simulink model "modelcompare"  (R2025b)
settings: Solver=VariableStepAuto  StartTime=0.0  StopTime=1296  RelTol=1e-3
(part 2 of 2)

== system modelcompare/Cooling Jacket Model4/Water to out ==
  Th : Inport
  mdot : Inport  Port=2
  Cpw : Inport  Port=3
  Mw : Inport  Port=4
  T_in : Inport  Port=5
  A : Inport  Port=6
  hw : Inport  Port=7
  Integrator2 : Integrator  InitialCondition=35
  MATLAB Function2 : MATLAB Function  TreatAsAtomicUnit=on
  Tout : Outport
  wires:
  Integrator2/1 -> Tout/1, MATLAB Function2/2(Tout)
  MATLAB Function2/1(dTout) -> Integrator2/1
  Th/1 -> MATLAB Function2/1(Th)
  T_in/1 -> MATLAB Function2/6(T_in)
  Mw/1 -> MATLAB Function2/3(Mw)
  mdot/1 -> MATLAB Function2/5(mdot)
  Cpw/1 -> MATLAB Function2/4(Cpw)
  A/1 -> MATLAB Function2/7(A)
  hw/1 -> MATLAB Function2/8(hw)

== system modelcompare/Cooling Jacket Model4/housing to water ==
  Ts : Inport
  k : Inport  Port=2
  d : Inport  Port=3
  Mh : Inport  Port=4
  Cph : Inport  Port=5
  A_sh : Inport  Port=6
  h : Inport  Port=7
  Tout : Inport  Port=8
  A_hw : Inport  Port=9
  Integrator1 : Integrator  InitialCondition=35
  MATLAB Function1 : MATLAB Function  TreatAsAtomicUnit=on
  Surface Temperature : Outport
  wires:
  MATLAB Function1/1(dTh) -> Integrator1/1
  k/1 -> MATLAB Function1/4(k)
  Ts/1 -> MATLAB Function1/1(Ts)
  Tout/1 -> MATLAB Function1/3(Tin)
  Integrator1/1 -> MATLAB Function1/2(Th), Surface Temperature/1
  d/1 -> MATLAB Function1/10(d_sh)
  Cph/1 -> MATLAB Function1/9(C_ph)
  Mh/1 -> MATLAB Function1/8(M_h)
  A_hw/1 -> MATLAB Function1/6(A_hw)
  A_sh/1 -> MATLAB Function1/5(A_sh)
  h/1 -> MATLAB Function1/7(h)

== matlab function modelcompare/Cooling Jacket Model2/MATLAB Function ==
  data: mdot input; h output; D input; CSA input; k input; f input; Pr input; Nu output; Re output; V output
function [h, Nu, Re, V]= fcn(mdot, D, CSA, k, f, Pr)
V = mdot/(1000*CSA);
Re = (V*1000*D)/0.00089;
Nu = ((f/8)*(Re-1000)*Pr)/(1+(12.7*(f/8)^0.5 * (Pr^(2/3) - 1)));
h = (Nu*k)/D;
end

== matlab function modelcompare/Battery Capacity/MATLAB Function ==
  data: Capacity output; energy input
function Capacity = fcn(energy)
    Capacity = energy/(12*3600);
end

== matlab function modelcompare/Battery Capacity1/MATLAB Function ==
  data: Capacity output; energy input
function Capacity = fcn(energy)
    Capacity = energy/(12*3600);
end

== matlab function modelcompare/Cooling Jacket Model1/MATLAB Function ==
  data: mdot input; h output; D input; CSA input; k input; f input; Pr input; Nu output; Re output; V output
function [h, Nu, Re, V]= fcn(mdot, D, CSA, k, f, Pr)
V = mdot/(1000*CSA);
Re = (V*1000*D)/0.00089;
Nu = ((f/8)*(Re-1000)*Pr)/(1+(12.7*(f/8)^0.5 * (Pr^(2/3) - 1)));
h = (Nu*k)/D;
end

== matlab function modelcompare/Cooling Jacket Model2/Stator to Housing/MATLAB Function ==
  data: Q_gen input; Ts input; dTs output; Th input; Ms input; Cps input; k input; A input; d input
function dTs = f1(Q_gen, Ts, Th, Ms, Cps, k, A, d)
    dTs = (Q_gen - (Ts - Th) * k * A / d) / (Ms * Cps);
end

== matlab function modelcompare/Cooling Jacket Model2/Water to out/MATLAB Function2 ==
  data: Th input; Tout input; Mw input; Cpw input; mdot input; T_in input; dTout output; A input; hw input
function dTout = f3(Th, Tout, Mw, Cpw, mdot, T_in, A, hw)
    q_from_housing = (Th - Tout) * hw * A;
    q_out = (Tout - T_in) * mdot * Cpw;
    dTout = ((q_from_housing - q_out)) / (Mw * Cpw);
end

== matlab function modelcompare/Cooling Jacket Model2/housing to water/MATLAB Function1 ==
  data: Ts input; Th input; Tin input; k input; A_sh input; A_hw input; dTh output; h input; M_h input; C_ph input; d_sh input
function dTh = f2(Ts, Th, Tin, k, A_sh, A_hw, h, M_h, C_ph, d_sh)
    dTh = ((k*A_sh*(Ts - Th)/d_sh) - h*A_hw*(Th - Tin)) / (M_h * C_ph);
end

== matlab function modelcompare/Cooling Jacket Model1/Stator to Housing/MATLAB Function ==
  data: Q_gen input; Ts input; dTs output; Th input; Ms input; Cps input; k input; A input; d input
function dTs = f1(Q_gen, Ts, Th, Ms, Cps, k, A, d)
    dTs = (Q_gen - (Ts - Th) * k * A / d) / (Ms * Cps);
end

== matlab function modelcompare/Cooling Jacket Model1/Water to out/MATLAB Function2 ==
  data: Th input; Tout input; Mw input; Cpw input; mdot input; T_in input; dTout output; A input; hw input
function dTout = f3(Th, Tout, Mw, Cpw, mdot, T_in, A, hw)
    q_from_housing = (Th - Tout) * hw * A;
    q_out = (Tout - T_in) * mdot * Cpw;
    dTout = ((q_from_housing - q_out)) / (Mw * Cpw);
end

== matlab function modelcompare/Cooling Jacket Model1/housing to water/MATLAB Function1 ==
  data: Ts input; Th input; Tin input; k input; A_sh input; A_hw input; dTh output; h input; M_h input; C_ph input; d_sh input
function dTh = f2(Ts, Th, Tin, k, A_sh, A_hw, h, M_h, C_ph, d_sh)
    dTh = ((k*A_sh*(Ts - Th)/d_sh) - h*A_hw*(Th - Tin)) / (M_h * C_ph);
end

== matlab function modelcompare/Pump Controller1/MATLAB Function ==
  data: StatorTemp input; mdot output; maximumFlowRate input; TempThreshold input
function mdot = fcn(StatorTemp, maximumFlowRate, TempThreshold)
if StatorTemp < 80 && StatorTemp > TempThreshold
    mdot = ((StatorTemp-TempThreshold)/(80 - TempThreshold))*maximumFlowRate;
elseif StatorTemp < TempThreshold
    mdot = 0;
else
    mdot = maximumFlowRate;
end
end

== matlab function modelcompare/Pump Controller1/MATLAB Function1 ==
  data: mdot input; power output; maxMdot input; maxcurrent input
function power = fcn(mdot, maxMdot, maxcurrent)
    power = (((4-maxcurrent)/(0-maxMdot))*(mdot - maxMdot) + maxcurrent)*12;
end

== matlab function modelcompare/Radiator1/MATLAB Function ==
  data: K input; h_wr output; D input; mdot input; A input
function h_wr = fcn(K, D, mdot, A)
Vm = mdot/(A * 24 * 1000);
Nu = 0.023 * (((1000*D*Vm)/0.001002)^0.8) * (6.9^0.4);
h_wr = (Nu * K)/D;
end

== matlab function modelcompare/Radiator1/MATLAB Function1 ==
  data: K input; h_ar output; D input; Va input
function h_ar = fcn(K, D, Va)
Nu = 0.664*((Va*D)/0.0000148)^0.5*(0.71)^0.33;
h_ar = (Nu * K)/D;
end

== matlab function modelcompare/Radiator1/Radiator to Air ==
  data: Trad input; Tair input; dTair output; A input; h input; v_air input; c_air input; m_air input; T_amb input; rho_air input
function dTair = f2(Trad, Tair, A, h, v_air, c_air, m_air, T_amb, rho_air)
    dTair = ((Trad - Tair) * h * A - (Tair - T_amb) * v_air * rho_air * A * c_air) / (m_air * c_air);
end

== matlab function modelcompare/Pump Controller/MATLAB Function1 ==
  data: mdot input; power output; maxMdot input; maxcurrent input
function power = fcn(mdot, maxMdot, maxcurrent)
    power = (((4-maxcurrent)/(0-maxMdot))*(mdot - maxMdot) + maxcurrent)*12;
end

== matlab function modelcompare/Radiator1/Water ==
  data: Tout_water input; T_in_water input; Trad input; dTout_water output; mdot_w input; c_w input; h_wr input; A_wr input; m_w_rad input
function dTout_water = f3(Tout_water, T_in_water, Trad, mdot_w, c_w, h_wr, A_wr, m_w_rad)
    dTout_water = ((T_in_water - Tout_water) * mdot_w * c_w - (Tout_water - Trad) * h_wr * A_wr) / (m_w_rad * c_w);
end

== matlab function modelcompare/Radiator1/Water to Radiator ==
  data: Trad input; Tair input; dTrad output; Tout_water input; h_wr input; A_wr input; h input; A input; m_rad input; c_rad input
function dTrad = f1(Trad, Tair, Tout_water, h_wr, A_wr, h, A, m_rad, c_rad)
    dTrad = ((Tout_water - Trad) * h_wr * A_wr - (Trad - Tair) * h * A) / (m_rad * c_rad);
end

== matlab function modelcompare/Battery Capacity3/MATLAB Function ==
  data: Capacity output; energy input
function Capacity = fcn(energy)
    Capacity = energy/(12*3600);
end

== matlab function modelcompare/Cooling Jacket Model4/MATLAB Function ==
  data: mdot input; h output; D input; CSA input; k input; f input; Pr input; Nu output; Re output; V output
function [h, Nu, Re, V]= fcn(mdot, D, CSA, k, f, Pr)
V = mdot/(1000*CSA);
Re = (V*1000*D)/0.00089;
Nu = ((f/8)*(Re-1000)*Pr)/(1+(12.7*(f/8)^0.5 * (Pr^(2/3) - 1)));
h = (Nu*k)/D;
end

== matlab function modelcompare/Cooling Jacket Model4/Stator to Housing/MATLAB Function ==
  data: Q_gen input; Ts input; dTs output; Th input; Ms input; Cps input; k input; A input; d input
function dTs = f1(Q_gen, Ts, Th, Ms, Cps, k, A, d)
    dTs = (Q_gen - (Ts - Th) * k * A / d) / (Ms * Cps);
end

== matlab function modelcompare/Cooling Jacket Model4/Water to out/MATLAB Function2 ==
  data: Th input; Tout input; Mw input; Cpw input; mdot input; T_in input; dTout output; A input; hw input
function dTout = f3(Th, Tout, Mw, Cpw, mdot, T_in, A, hw)
    q_from_housing = (Th - Tout) * hw * A;
    q_out = (Tout - T_in) * mdot * Cpw;
    dTout = ((q_from_housing - q_out)) / (Mw * Cpw);
end

== matlab function modelcompare/Cooling Jacket Model4/housing to water/MATLAB Function1 ==
  data: Ts input; Th input; Tin input; k input; A_sh input; A_hw input; dTh output; h input; M_h input; C_ph input; d_sh input
function dTh = f2(Ts, Th, Tin, k, A_sh, A_hw, h, M_h, C_ph, d_sh)
    dTh = ((k*A_sh*(Ts - Th)/d_sh) - h*A_hw*(Th - Tin)) / (M_h * C_ph);
end

== matlab function modelcompare/Pump Controller/MATLAB Function ==
  data: mdot output
function mdot = fcn()

    mdot = 0.15;

end

== matlab function modelcompare/Pump Controller3/MATLAB Function1 ==
  data: mdot input; power output; maxMdot input; maxcurrent input
function power = fcn(mdot, maxMdot, maxcurrent)
    power = (((4-maxcurrent)/(0-maxMdot))*(mdot - maxMdot) + maxcurrent)*12;
end

== matlab function modelcompare/Radiator3/MATLAB Function ==
  data: K input; h_wr output; D input; mdot input; A input
function h_wr = fcn(K, D, mdot, A)
Vm = mdot/(A * 24 * 1000);
Nu = 0.023 * (((1000*D*Vm)/0.001002)^0.8) * (6.9^0.4);
h_wr = (Nu * K)/D;
end

== matlab function modelcompare/Radiator3/MATLAB Function1 ==
  data: K input; h_ar output; D input; Va input
function h_ar = fcn(K, D, Va)
Nu = 0.664*((Va*D)/0.0000148)^0.5*(0.71)^0.33;
h_ar = (Nu * K)/D;
end

== matlab function modelcompare/Radiator3/Radiator to Air ==
  data: Trad input; Tair input; dTair output; A input; h input; v_air input; c_air input; m_air input; T_amb input; rho_air input
function dTair = f2(Trad, Tair, A, h, v_air, c_air, m_air, T_amb, rho_air)
    dTair = ((Trad - Tair) * h * A - (Tair - T_amb) * v_air * rho_air * A * c_air) / (m_air * c_air);
end

== matlab function modelcompare/Radiator3/Water ==
  data: Tout_water input; T_in_water input; Trad input; dTout_water output; mdot_w input; c_w input; h_wr input; A_wr input; m_w_rad input
function dTout_water = f3(Tout_water, T_in_water, Trad, mdot_w, c_w, h_wr, A_wr, m_w_rad)
    dTout_water = ((T_in_water - Tout_water) * mdot_w * c_w - (Tout_water - Trad) * h_wr * A_wr) / (m_w_rad * c_w);
end

== matlab function modelcompare/Radiator/MATLAB Function ==
  data: K input; h_wr output; D input; mdot input; A input
function h_wr = fcn(K, D, mdot, A)
Vm = mdot/(A * 24 * 1000);
Nu = 0.023 * (((1000*D*Vm)/0.001002)^0.8) * (6.9^0.4);
h_wr = (Nu * K)/D;
end

== matlab function modelcompare/Radiator3/Water to Radiator ==
  data: Trad input; Tair input; dTrad output; Tout_water input; h_wr input; A_wr input; h input; A input; m_rad input; c_rad input
function dTrad = f1(Trad, Tair, Tout_water, h_wr, A_wr, h, A, m_rad, c_rad)
    dTrad = ((Tout_water - Trad) * h_wr * A_wr - (Trad - Tair) * h * A) / (m_rad * c_rad);
end

== matlab function modelcompare/Radiator/Water to Radiator ==
  data: Trad input; Tair input; dTrad output; Tout_water input; h_wr input; A_wr input; h input; A input; m_rad input; c_rad input
function dTrad = f1(Trad, Tair, Tout_water, h_wr, A_wr, h, A, m_rad, c_rad)
    dTrad = ((Tout_water - Trad) * h_wr * A_wr - (Trad - Tair) * h * A) / (m_rad * c_rad);
end

== matlab function modelcompare/Radiator/Radiator to Air ==
  data: Trad input; Tair input; dTair output; A input; h input; v_air input; c_air input; m_air input; T_amb input; rho_air input
function dTair = f2(Trad, Tair, A, h, v_air, c_air, m_air, T_amb, rho_air)
    dTair = ((Trad - Tair) * h * A - (Tair - T_amb) * v_air * rho_air * A * c_air) / (m_air * c_air);
end

== matlab function modelcompare/Radiator/Water ==
  data: Tout_water input; T_in_water input; Trad input; dTout_water output; mdot_w input; c_w input; h_wr input; A_wr input; m_w_rad input
function dTout_water = f3(Tout_water, T_in_water, Trad, mdot_w, c_w, h_wr, A_wr, m_w_rad)
    dTout_water = ((T_in_water - Tout_water) * mdot_w * c_w - (Tout_water - Trad) * h_wr * A_wr) / (m_w_rad * c_w);
end

== matlab function modelcompare/Radiator/MATLAB Function1 ==
  data: K input; h_ar output; D input; Va input
function h_ar = fcn(K, D, Va)
Nu = 0.664*((Va*D)/0.0000148)^0.5*(0.71)^0.33;
h_ar = (Nu * K)/D;
end
